simulink library "aerolibconvert"  (Simulink 5.0)
values from neighbouring files (symbols this model uses):
  s = aeroliblist    [asbhelp.m]
undefined symbols (not defined in the file or in its folder): bias, slope
settings Model: Creator=sgage  LastModifiedBy=sgage  ExtModeAutoUpdateStatusClock=off

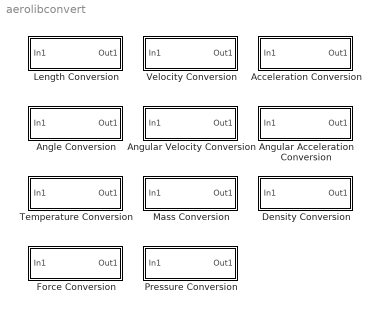
== system aerolibconvert ==
  Acceleration Conversion : Subsystem  mask(Acceleration Conversion){IU=ft/s^2, OU=m/s^2}
      mask prompts: IU "Initial units:"; OU "Final units:"
      mask help: Convert units of input signal to desired output units.
      mask init:
      | aeroicon('aeroblkconversion');
      | [ports,slope,bias] = aeroicon('aeroblkconversion','icon');
      | [xp,yp]=aeroimage('unitconv');
      mask Help: web(asbhelp);
      mask StyleString: popup(ft/s^2|m/s^2|km/s^2|in/s^2|km/h-s|mph/s),popup(ft/s^2|m/s^2|km/s^2|in/s^2|km/h-s|mph/s)
      mask Display:
      | port_label(ports(1).type,ports(1).port,ports(1).txt,'texmode','on');
      | port_label(ports(2).type,ports(2).port,ports(2).txt,'texmode','on');
      | patch(xp,yp)
  Angle Conversion : Subsystem  mask(Angle Conversion){IU=deg, OU=rad}
      mask prompts: IU "Initial units:"; OU "Final units:"
      mask help: Convert units of input signal to desired output units.
      mask init:
      | aeroicon('aeroblkconversion');
      | [ports,slope,bias] = aeroicon('aeroblkconversion','icon');
      | [xp,yp]=aeroimage('unitconv');
      mask Help: web(asbhelp);
      mask StyleString: popup(deg|rad|rev),popup(deg|rad|rev)
      mask Display:
      | port_label(ports(1).type,ports(1).port,ports(1).txt);
      | port_label(ports(2).type,ports(2).port,ports(2).txt);
      | patch(xp,yp)
  Angular Acceleration Conversion : Subsystem  mask(Angular Acceleration Conversion){IU=deg/s^2, OU=rad/s^2}
      mask prompts: IU "Initial units:"; OU "Final units:"
      mask help: Convert units of input signal to desired output units.
      mask init:
      | aeroicon('aeroblkconversion');
      | [ports,slope,bias] = aeroicon('aeroblkconversion','icon');
      | [xp,yp]=aeroimage('unitconv');
      mask Help: web(asbhelp);
      mask StyleString: popup(deg/s^2|rad/s^2|rpm/s),popup(deg/s^2|rad/s^2|rpm/s)
      mask Display:
      | port_label(ports(1).type,ports(1).port,ports(1).txt,'texmode','on');
      | port_label(ports(2).type,ports(2).port,ports(2).txt,'texmode','on');
      | patch(xp,yp)
  Angular Velocity Conversion : Subsystem  mask(Angular Velocity Conversion){IU=deg/s, OU=rad/s}
      mask prompts: IU "Initial units:"; OU "Final units:"
      mask help: Convert units of input signal to desired output units.
      mask init:
      | aeroicon('aeroblkconversion');
      | [ports,slope,bias] = aeroicon('aeroblkconversion','icon');
      | [xp,yp]=aeroimage('unitconv');
      mask Help: web(asbhelp);
      mask StyleString: popup(deg/s|rad/s|rpm),popup(deg/s|rad/s|rpm)
      mask Display:
      | port_label(ports(1).type,ports(1).port,ports(1).txt);
      | port_label(ports(2).type,ports(2).port,ports(2).txt);
      | patch(xp,yp)
  Density Conversion : Subsystem  mask(Density Conversion){IU=lbm/ft^3, OU=kg/m^3}
      mask prompts: IU "Initial units:"; OU "Final units:"
      mask help: Convert units of input signal to desired output units.
      mask init:
      | aeroicon('aeroblkconversion');
      | [ports,slope,bias] = aeroicon('aeroblkconversion','icon');
      | [xp,yp]=aeroimage('unitconv');
      mask Help: web(asbhelp);
      mask StyleString: popup(lbm/ft^3|kg/m^3|slug/ft^3|lbm/in^3),popup(lbm/ft^3|kg/m^3|slug/ft^3|lbm/in^3)
      mask Display:
      | port_label(ports(1).type,ports(1).port,ports(1).txt,'texmode','on');
      | port_label(ports(2).type,ports(2).port,ports(2).txt,'texmode','on');
      | patch(xp,yp)
  Force Conversion : Subsystem  mask(Force Conversion){IU=lbf, OU=N}
      mask prompts: IU "Initial units:"; OU "Final units:"
      mask help: Convert units of input signal to desired output units.
      mask init:
      | aeroicon('aeroblkconversion');
      | [ports,slope,bias] = aeroicon('aeroblkconversion','icon');
      | [xp,yp]=aeroimage('unitconv');
      mask Help: web(asbhelp);
      mask StyleString: popup(lbf|N),popup(lbf|N)
      mask Display:
      | port_label(ports(1).type,ports(1).port,ports(1).txt);
      | port_label(ports(2).type,ports(2).port,ports(2).txt);
      | patch(xp,yp)
  Length Conversion : Subsystem  mask(Length Conversion){IU=ft, OU=m}
      mask prompts: IU "Initial units:"; OU "Final units:"
      mask help: Convert units of input signal to desired output units.
      mask init:
      | aeroicon('aeroblkconversion');
      | [ports,slope,bias] = aeroicon('aeroblkconversion','icon');
      | [xp,yp]=aeroimage('unitconv');
      mask Help: web(asbhelp);
      mask StyleString: popup(ft|m|km|in|mi|naut mi),popup(ft|m|km|in|mi|naut mi)
      mask Display:
      | port_label(ports(1).type,ports(1).port,ports(1).txt);
      | port_label(ports(2).type,ports(2).port,ports(2).txt);
      | patch(xp,yp)
  Mass Conversion : Subsystem  mask(Mass Conversion){IU=lbm, OU=kg}
      mask prompts: IU "Initial units:"; OU "Final units:"
      mask help: Convert units of input signal to desired output units.
      mask init:
      | aeroicon('aeroblkconversion');
      | [ports,slope,bias] = aeroicon('aeroblkconversion','icon');
      | [xp,yp]=aeroimage('unitconv');
      mask Help: web(asbhelp);
      mask StyleString: popup(lbm|kg|slug),popup(lbm|kg|slug)
      mask Display:
      | port_label(ports(1).type,ports(1).port,ports(1).txt);
      | port_label(ports(2).type,ports(2).port,ports(2).txt);
      | patch(xp,yp)
  Pressure Conversion : Subsystem  mask(Pressure Conversion){IU=psi, OU=Pa}
      mask prompts: IU "Initial units:"; OU "Final units:"
      mask help: Convert units of input signal to desired output units.
      mask init:
      | aeroicon('aeroblkconversion');
      | [ports,slope,bias] = aeroicon('aeroblkconversion','icon');
      | [xp,yp]=aeroimage('unitconv');
      mask Help: web(asbhelp);
      mask StyleString: popup(psi|Pa|psf|atm),popup(psi|Pa|psf|atm)
      mask Display:
      | port_label(ports(1).type,ports(1).port,ports(1).txt);
      | port_label(ports(2).type,ports(2).port,ports(2).txt);
      | patch(xp,yp)
  Temperature Conversion : Subsystem  mask(Temperature Conversion){IU=R, OU=K}
      mask prompts: IU "Initial units:"; OU "Final units:"
      mask help: Convert units of input signal to desired output units.
      mask init:
      | aeroicon('aeroblkconversion');
      | [ports,slope,bias] = aeroicon('aeroblkconversion','icon');
      | [xp,yp]=aeroimage('unitconv');
      mask Help: web(asbhelp);
      mask StyleString: popup(K|F|C|R),popup(K|F|C|R)
      mask Display:
      | port_label(ports(1).type,ports(1).port,ports(1).txt);
      | port_label(ports(2).type,ports(2).port,ports(2).txt);
      | patch(xp,yp)
  Velocity Conversion : Subsystem  mask(Velocity Conversion){IU=ft/s, OU=m/s}
      mask prompts: IU "Initial units:"; OU "Final units:"
      mask help: Convert units of input signal to desired output units.
      mask init:
      | aeroicon('aeroblkconversion');
      | [ports,slope,bias] = aeroicon('aeroblkconversion','icon');
      | [xp,yp]=aeroimage('unitconv');
      mask Help: web(asbhelp);
      mask StyleString: popup(ft/s|m/s|km/s|in/s|km/h|mph|kts),popup(ft/s|m/s|km/s|in/s|km/h|mph|kts)
      mask Display:
      | port_label(ports(1).type,ports(1).port,ports(1).txt);
      | port_label(ports(2).type,ports(2).port,ports(2).txt);
      | patch(xp,yp)

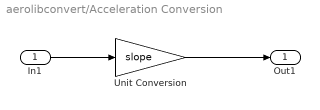
== system aerolibconvert/Acceleration Conversion ==
  In1 : Inport
  Unit Conversion : Gain  Gain=slope  SaturateOnIntegerOverflow=on
  Out1 : Outport
  wires:
  In1/1 -> Unit Conversion/1
  Unit Conversion/1 -> Out1/1

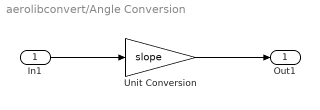
== system aerolibconvert/Angle Conversion ==
  In1 : Inport
  Unit Conversion : Gain  Gain=slope  SaturateOnIntegerOverflow=on
  Out1 : Outport
  wires:
  Unit Conversion/1 -> Out1/1
  In1/1 -> Unit Conversion/1

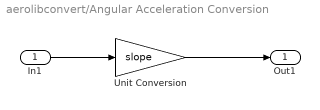
== system aerolibconvert/Angular Acceleration Conversion ==
  In1 : Inport
  Unit Conversion : Gain  Gain=slope  SaturateOnIntegerOverflow=on
  Out1 : Outport
  wires:
  Unit Conversion/1 -> Out1/1
  In1/1 -> Unit Conversion/1

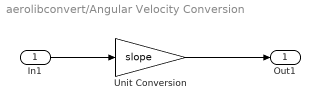
== system aerolibconvert/Angular Velocity Conversion ==
  In1 : Inport
  Unit Conversion : Gain  Gain=slope  SaturateOnIntegerOverflow=on
  Out1 : Outport
  wires:
  In1/1 -> Unit Conversion/1
  Unit Conversion/1 -> Out1/1

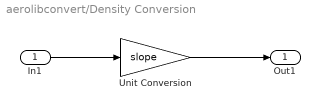
== system aerolibconvert/Density Conversion ==
  In1 : Inport
  Unit Conversion : Gain  Gain=slope  SaturateOnIntegerOverflow=on
  Out1 : Outport
  wires:
  Unit Conversion/1 -> Out1/1
  In1/1 -> Unit Conversion/1

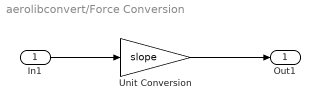
== system aerolibconvert/Force Conversion ==
  In1 : Inport
  Unit Conversion : Gain  Gain=slope  SaturateOnIntegerOverflow=on
  Out1 : Outport
  wires:
  In1/1 -> Unit Conversion/1
  Unit Conversion/1 -> Out1/1

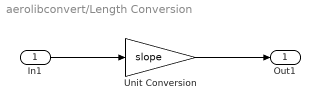
== system aerolibconvert/Length Conversion ==
  In1 : Inport
  Unit Conversion : Gain  Gain=slope  SaturateOnIntegerOverflow=on
  Out1 : Outport
  wires:
  In1/1 -> Unit Conversion/1
  Unit Conversion/1 -> Out1/1

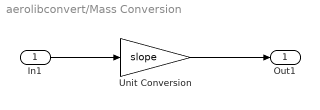
== system aerolibconvert/Mass Conversion ==
  In1 : Inport
  Unit Conversion : Gain  Gain=slope  SaturateOnIntegerOverflow=on
  Out1 : Outport
  wires:
  Unit Conversion/1 -> Out1/1
  In1/1 -> Unit Conversion/1

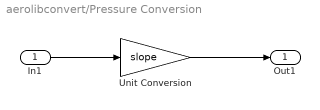
== system aerolibconvert/Pressure Conversion ==
  In1 : Inport
  Unit Conversion : Gain  Gain=slope  SaturateOnIntegerOverflow=on
  Out1 : Outport
  wires:
  In1/1 -> Unit Conversion/1
  Unit Conversion/1 -> Out1/1

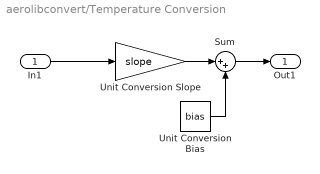
== system aerolibconvert/Temperature Conversion ==
  In1 : Inport
  Sum : Sum  Inputs=|++  SaturateOnIntegerOverflow=on  InputSameDT=on
  Unit Conversion Bias : Constant  Value=bias  ShowAdditionalParam=on
  Unit Conversion Slope : Gain  Gain=slope  SaturateOnIntegerOverflow=on
  Out1 : Outport
  wires:
  In1/1 -> Unit Conversion Slope/1
  Unit Conversion Slope/1 -> Sum/1
  Sum/1 -> Out1/1
  Unit Conversion Bias/1 -> Sum/2

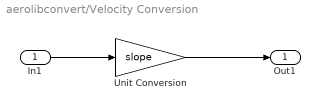
== system aerolibconvert/Velocity Conversion ==
  In1 : Inport
  Unit Conversion : Gain  Gain=slope  SaturateOnIntegerOverflow=on
  Out1 : Outport
  wires:
  Unit Conversion/1 -> Out1/1
  In1/1 -> Unit Conversion/1
